simulink subsystem "HallSensor2022"  (R2023a)
settings: Solver=VariableStepAuto  StartTime=0.0  StopTime=10.0  RelTol=1e-3
settings Model: Creator=mrrom  LastModifiedBy=romav

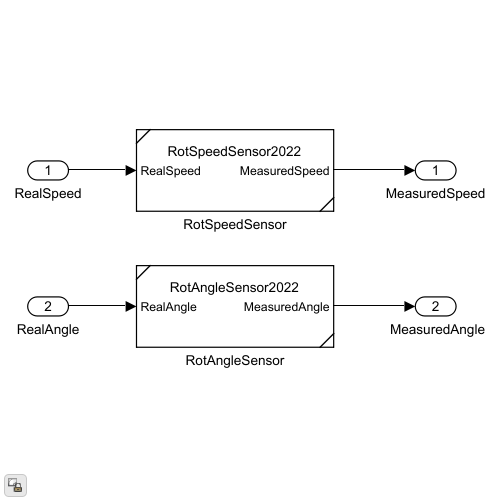
[thumbnail: Simulink's stored preview of the top-level diagram]
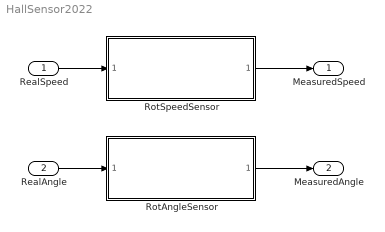
== system HallSensor2022 ==
  RealSpeed : Inport
  RealAngle : Inport  Port=2
  RotAngleSensor : Subsystem  ReferencedSubsystem=RotAngleSensor2022
  RotSpeedSensor : Subsystem  ReferencedSubsystem=RotSpeedSensor2022
  MeasuredSpeed : Outport
  " MeasuredAngle" : Outport  Port=2
  wires:
  RealAngle/1 -> RotAngleSensor/1
  RotAngleSensor/1 -> " MeasuredAngle"/1
  RealSpeed/1 -> RotSpeedSensor/1
  RotSpeedSensor/1 -> MeasuredSpeed/1
